simulink library "vmc"  (R2021b)
settings: Solver=VariableStepAuto  StartTime=0.0  StopTime=10.0  RelTol=1e-3
undefined symbols (not defined in the file or in its folder): AVMC_ACCDeltaTqIGain_X_kph, AVMC_ACCDeltaTqIGain_Y_mps2, AVMC_ACCDeltaTqPGain_X_kph, AVMC_ACCDeltaTqPGain_Y_kph, AVMC_ACCLongSteadyCtrl_X_kph, AVMC_AggressJerkPCT4AT_X_kph, AVMC_AggressJerkPCT_X_kph, AVMC_AggressLimitPCT4AT_X_kph, AVMC_AggressLimitPCT_X_kph, AVMC_CCLongSteadyCtrl_X_kph, AVMC_DISCDeltaTqIGain_X_kph, AVMC_DISCDeltaTqIGain_Y_mps2, AVMC_DISCDeltaTqPGain_X_kph, AVMC_DISCDeltaTqPGain_Y_kph, AVMC_DISCTrunAccJerk_X_s, AVMC_DISCTrunAccLimit_X_s, AVMC_ESCRegenOut_X_kph, AVMC_ESCRegenOut_Y_Deg, AVMC_ESCRegenOutEnSpd_X_Deg, AVMC_ISOAccLimit_X_mps, AVMC_ISODecLimit_X_mps, AVMC_ISOJerk_X_mps, AVMC_LatESCRegenOut_X_kph, AVMC_LatESCRegenOut_Y_Deg, AVMC_LongAccDeadZone_X_kph, AVMC_LongAccFiltTsforP2_X_Gps, AVMC_MCPresBaseTq_X_bar, AVMC_MSALongSteadyCtrl_X_kph, AVMC_MSAPedalOvrd2_X_kph, AVMC_MSAPedalOvrd_X_kph, AVMC_MSASpdBand_X_kph, AVMC_MSATqDownEndTq_X_kph, AVMC_MSATqDownTime_X_kph, AVMC_OPDDisSlideRate_X_Deg, AVMC_RDCDetectTime_X_kph, AVMC_RDCDetectTime_Y_pct, AVMC_RDCEnSlideRate_X_Deg, AVMC_RearWhlTqRatio_X_Nm, AVMC_RearWhlTqRatio_Y_gps, AVMC_RearWhlTqSlipGain_X_rat, AVMC_RearWhlTqSlipGain_Y_kph, AVMC_RearWhlTqSTRGGain_X_deg, AVMC_RearWhlTqSTRGGain_Y_kph, AVMC_RWSRrTSA2RWSPos_X_deg, AVMC_RWSSAS2FrtTSA_X_deg, AVMC_RWSVehSPD2RWSCoef_X_kph, AVMC_SoftJerkPCT_X_kph, AVMC_SoftLimitPCT_X_kph, AVMC_StESCYaw_X_kph, AVMC_StESCYaw_Y_Deg, AVMC_StESCYawCom_X_kph, AVMC_StESCYawCom_Y_Gps, AVMC_TMSpdBaseTq_X_rpm, AVMC_VehHoldBDecMap_X_kph, AVMC_VehHoldDecCtrlTime_X_kph, AVMC_VehHoldMCPPass_X_deg, C_TASK_10MS_S, C_TASK_5MS_S, DEG2RAD, ENUM_ACCAVAIL_AVAILABLE ... (+409)
libraries: hcu_lib x74, simulink x68, simulink_extras x3, $bdroot x2
(part 10 of 15)

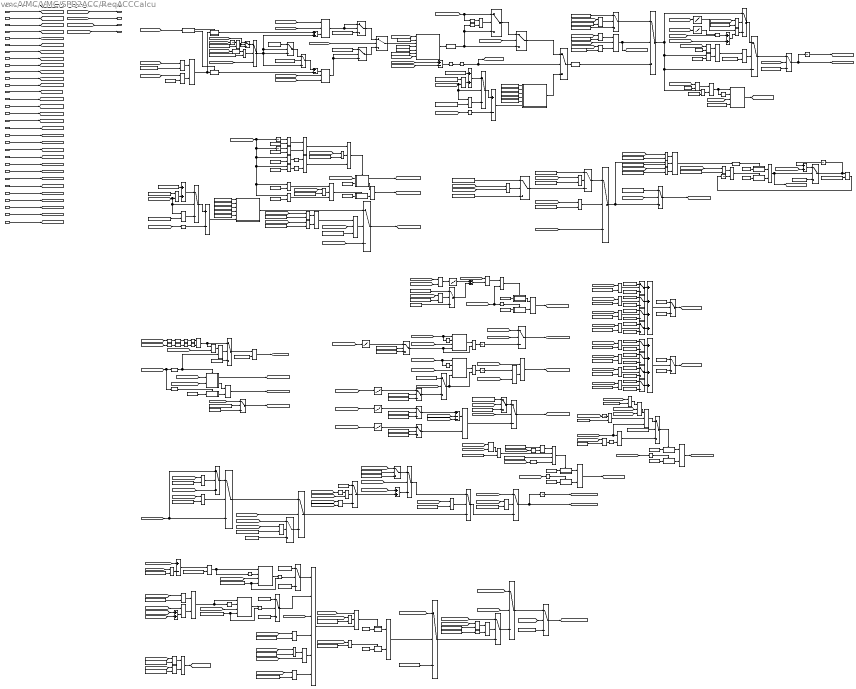
== system vmc/VMC/VMC/SPD2ACC/ReqACCCalcu ==
  note: FVT Soft Stop Control
      | (Send Hold Command after Reach H Time or ESC Standstill)
  note: Follow DISC Hold Time
      | (Avoid arbitrate error since CAN Signal sample time difference)
  note: Smooth Switch
      | (A, B-Pedal & REGEN to DISC)
  note: Required Acceleration for ESC
  note: Actual Required Acceleration
  note: DISC Required Acceleration
  note: Acceleration Arbitration
  note: ACC Speed Control
  note: Minimum Resolution
      | (Avoid too small command calculated from ISO Limit)
  note: Constant Speed Control
  note: Vehicle Hold Judgement and Command
  note: ACC Constant Speed Control
  note: ACC Constant Speed Control Judgement
  VVMC_AccCalcuPID_mps2 : Inport
  VVMC_ISOJerkLimit_mps3 : Inport  Port=2
  VVMC_JerkPCT_pct : Inport  Port=3
  VVMC_ISOAccLimit_mps2 : Inport  Port=4
  VVMC_ISODecLimit_mps2 : Inport  Port=5
  VVMC_SPD2ACCAct_flg : Inport  Port=6
  VVMC_SafetyCtrl_flg : Inport  Port=7
  VINP_ACCRequiredAccel_mps2 : Inport  Port=8
  VVMC_FeatArbitrSta_enum : Inport  Port=9
  VINP_ADASACCSta_enum : Inport  Port=10
  VVMC_MeterIndSpeedForCalcu_kph : Inport  Port=11
  VVMC_FeatReqSpd_kph : Inport  Port=12
  task_time_s : Inport  Port=13
  VINP_VehSpeed_kph : Inport  Port=14
  VVMC_LongAcc_Gps : Inport  Port=15
  VINP_ESCADASSta_enum : Inport  Port=16
  VVMC_LastADASWhlTqReq_Nm : Inport  Port=17
  VTQD_RrEDUAvailBrkRgnTq_Nm : Inport  Port=18
  VVMC_ACCVehHoldReq_flg : Inport  Port=19
  VVMC_EstSlope_Deg : Inport  Port=20
  VVMC_LongAccDeadZone_Gps : Inport  Port=21
  VTQD_FrEDUAvailBrkRgnTq_Nm : Inport  Port=22
  VVMC_ACCLowSpdTqCtrl_flg : Inport  Port=23
  VDSC_DISCTurn_flg : Inport  Port=24
  VINP_GRADE_Deg : Inport  Port=25
  VINP_LFWhlRotDir_enum : Inport  Port=26
  VINP_LRWhlRotDir_enum : Inport  Port=27
  VINP_RFWhlRotDir_enum : Inport  Port=28
  VINP_RRWhlRotDir_enum : Inport  Port=29
  VVMC_ACCObjDist_m : Inport  Port=30
  VINP_MCPressure_bar : Inport  Port=31
  VVMC_AccelTurnHold_flg : Inport  Port=32
  AND : Logic  Operator=OR  AllPortsSameDT=off  OutDataTypeStr=boolean
  AND{1,5..6,8..12,15} (9 alike) : Logic  AllPortsSameDT=off  OutDataTypeStr=boolean
  AND18 : Logic  Inputs=4  AllPortsSameDT=off  OutDataTypeStr=boolean
  AND2 : Logic  Inputs=3  AllPortsSameDT=off  OutDataTypeStr=boolean
  AND3 : Logic  Inputs=3  AllPortsSameDT=off  OutDataTypeStr=boolean
  AND4 : Logic  Inputs=3  AllPortsSameDT=off  OutDataTypeStr=boolean
  AND7 : Logic  Operator=OR  AllPortsSameDT=off  OutDataTypeStr=boolean
  Abs{,1..4} (5 alike) : Abs
  Add{,2,5,7,9} (5 alike) : Sum  Inputs=+-
  Add{1,3..4,6,8,11,14..15} (8 alike) : Sum
  Add10 : Sum  Inputs=+--
  Add12 : Sum  Inputs=++++
  Add13 : Sum  Inputs=++++
  CMDRepeat : Stateflow chart  TreatAsAtomicUnit=on
      settings: PortSchema="{\"entries\":[{\"content\":{\"sides\":[{\"content\":{\"connectorIds\":[\"In1\",\"In3\",\"In2\",\"In4\",\"In5\",\"In6\",\"In7\"]},\"type\":\"ConnectorPlacement.EquallySpacedRectSide\",\"uuid\":\"905b82c5-26d0-4d78-9cc9-ade9518b6cb1\"},{\"content\":{\"connectorIds\":[\"Out1\"],\"side\":\"RIGHT\"},\"type\":\"ConnectorPlacement.EquallySpacedRectSide\",\"uuid\":\"7321c4d8-dca0-41f9-ac80-faa74e816847\"},{\"content\":{\"connectorIds\":[],\"side\":\"TOP\"},\"type\":\"ConnectorPlacement.EquallySpacedRectSide\",\"uuid\":\"61a83612-f0ae-4eca-a4ee-e5180dc2049c\"}]},\"type\":\"ConnectorPlacement.EquallySpacedConnector\",\"uuid\":\"6863a8ab-8f7f-41d7-93f0-c1bbef1d5e3d\"}],\"packageUris\":[\"http://schema.mathworks.com/mf0/Connector/R2020b\"],\"version\":\"1.0\"}"
  Cast To Single{,1..2,7} (4 alike) : DataTypeConversion  OutDataTypeStr=single
  Constant : Constant  Value=pct
  Constant{1,7,19,27,34,39..40,42,44..45,49,64,66..68,78..79,81,89..93,95,112,115,125,127,129,131,139,141,143,145,157,163} (36 alike) : Constant  Value=ZERO_FLOAT
  Constant{10..12,17,20,32} (6 alike) : Constant  Value=ENUM_FEATARBITRSTA_DISC
  Constant100 : Constant  Value=KVMC_VehHoldDecCtrlBSlope4ATH_mps3
  Constant101 : Constant  Value=KVMC_ReqBrkJoinWaitTime_s
  Constant{50,52,70,102,106,108,134,148,150,153} (10 alike) : Constant  Value=FALSE
  Constant{48,51,69,94,97,103,107,109,111,133,147,154,161} (13 alike) : Constant  Value=TRUE
  Constant104 : Constant  Value=KVMC_AGSVReqAccel_mps2
  Constant105 : Constant  Value=KVMC_ReqBrkJoinWaitTime_s
  Constant110 : Constant  Value=KVMC_DISCTurnAccCtrl_flg
  Constant113 : Constant  Value=KVMC_DISCTurnAccSoftTime_s
  Constant114 : Constant  Value=KVMC_DISCTurnAccSoftTime_s
  Constant{117,122..124} (4 alike) : Constant  Value=ENUM_WheelRotDir_STANDSTILL
  Constant118 : Constant  Value=KVMC_VehHoldDelayHEndSW_flg
  Constant119 : Constant  Value=KVMC_VehHoldDist_m
  Constant121 : Constant  Value=KVMC_VehHoldDecCtrlCalSW2_flg
  Constant{30,126,128,130,132,140,142,144,146} (9 alike) : Constant  Value=ONE_FLOAT
  Constant{6,13,33,55,61} (5 alike) : Constant  Value=ENUM_FEATARBITRSTA_ACC
  Constant{135..138} (4 alike) : Constant  Value=ENUM_WheelRotDir_BACKWARD
  Constant14 : Constant  Value=KVMC_SpdCtrlEnBand_kph
  Constant149 : Constant  Value=KVMC_UpHillHoldDelayDeg_deg
  Constant15 : Constant  Value=KVMC_VehHoldDecCtrlBDec_mps2
  Constant151 : Constant  Value=KVMC_VehHoldDecCtrlBSlope_mps3
  Constant152 : Constant  Value=ENUM_FEATARBITRSTA_AEB
  Constant155 : Constant  Value=KVMC_DecCreepTq_Nm
  Constant156 : Constant  Value=KVMC_CreepTqMCP_bar
  Constant16 : Constant  Value=KVMC_Veh2MeterSpdFactor_enum
  Constant162 : Constant  Value=KVMC_VehHoldDecCtrlHTime2_s
  Constant18 : Constant  Value=KVMC_FollowDISCHoldTime_s
  Constant2 : Constant  Value=KVMC_CMDCycleTime_s
  Constant{5,8,21,56} (4 alike) : Constant  Value=ENUM_FEATARBITRSTA_ACCDISC
  Constant22 : Constant  Value=KVMC_AccelPos2NegSWC_flg
  Constant23 : Constant  Value=KVMC_Veh2MeterSpdOffset_enum
  Constant24 : Constant  Value=KVMC_SpdCtrlDisBand_kph
  Constant25 : Constant  Value=MINUSONE_FLOAT
  Constant26 : Constant  Value=KVMC_SpdCtrlReqAccel_mps2
  Constant28 : Constant  Value=KVMC_Veh2MeterSpdLoFactor_enum
  Constant29 : Constant  Value=KVMC_VehHoldSpd_kph
  Constant3 : Constant  Value=ZERO_INT
  Constant31 : Constant  Value=KVMC_VehHoldDecel_mps2
  Constant35 : Constant  Value=KVMC_SPD2ACCLastAccelSourceSW_flg
  Constant36 : Constant  Value=ENUM_ESCADASSTA_VEHASTANDSTILL
  Constant37 : Constant  Value=KVMC_GravityValue_mps2
  Constant{38,84..85,87,96} (5 alike) : Constant  Value=KVMC_VehHoldDecCtrlCalSW_flg
  Constant4 : Constant  Value=KVMC_CMDRepeatTime_enum
  Constant41 : Constant  Value=KVMC_GravityValue_mps2
  Constant43 : Constant  Value=KVMC_AccelCtrlTqLowerLimit_Nm
  Constant46 : Constant  Value=KVMC_SprtAccelCMDSW_flg
  Constant47 : Constant  Value=KVMC_TqAccelCtrlBand_mps2
  Constant53 : Constant  Value=KVMC_ReqAccelLowerLimit_mps2
  Constant54 : Constant  Value=KVMC_ReqDecelLowerLimit_mps2
  Constant57 : Constant  Value=KVMC_SpdCtrlEnBand_kph
  Constant58 : Constant  Value=KVMC_Veh2MeterSpdFactor_enum
  Constant59 : Constant  Value=KVMC_Veh2MeterSpdOffset_enum
  Constant60 : Constant  Value=KVMC_SpdCtrlDisBand_kph
  Constant62 : Constant  Value=MINUSONE_FLOAT
  Constant63 : Constant  Value=KVMC_SpdCtrlReqAccel_mps2
  Constant65 : Constant  Value=KVMC_Veh2MeterSpdLoFactor_enum
  Constant71 : Constant  Value=KVMC_ACCSpdCtrlSW_flg
  Constant72 : Constant  Value=ENUM_ADASACCSTA_OVERRIDE
  Constant73 : Constant  Value=ENUM_ADASACCSTA_OVERRIDE
  Constant74 : Constant  Value=KVMC_VehHoldDecCtrl_flg
  Constant75 : Constant  Value=KVMC_VehHoldDecCtrlBTime_s
  Constant76 : Constant  Value=KVMC_VehHoldDecCtrlBDec_mps2
  Constant77 : Constant  Value=KVMC_GravityValue_mps2
  Constant80 : Constant  Value=KVMC_VehHoldDecCtrlBTime_s
  Constant82 : Constant  Value=KVMC_CallBrkJoinSpd_kph
  Constant83 : Constant  Value=KVMC_VehHoldDecCtrlHTime_s
  Constant86 : Constant  Value=ENUM_ADASACCSTA_ACTIVE
  Constant88 : Constant  Value=KVMC_VehHoldDecCtrlGFBSW_flg
  Constant9 : Constant  Value=ENUM_ADASACCSTA_OVERRIDE
  Constant98 : Constant  Value=KVMC_AccelTurnHoldDecCtrl2_flg
  Constant99 : Constant  Value=ENUM_ADASACCSTA_ACTIVE
  ConstantSpeedControl : Stateflow chart  TreatAsAtomicUnit=on
      settings: PortSchema="{\"entries\":[{\"content\":{\"sides\":[{\"content\":{\"connectorIds\":[\"In2\",\"In3\",\"In4\",\"In5\",\"In6\",\"In1\"]},\"type\":\"ConnectorPlacement.EquallySpacedRectSide\",\"uuid\":\"931d4d55-b643-4b97-a7aa-1deb2b509e83\"},{\"content\":{\"connectorIds\":[\"Out1\"],\"side\":\"RIGHT\"},\"type\":\"ConnectorPlacement.EquallySpacedRectSide\",\"uuid\":\"f2f28b13-6937-4f35-b44e-683edec0d4ba\"},{\"content\":{\"connectorIds\":[],\"side\":\"TOP\"},\"type\":\"ConnectorPlacement.EquallySpacedRectSide\",\"uuid\":\"e2886b86-de2a-4a68-b05f-bfb0f2051baf\"}]},\"type\":\"ConnectorPlacement.EquallySpacedConnector\",\"uuid\":\"cece4c76-e980-42e8-adab-da09fec387c1\"}],\"packageUris\":[\"http://schema.mathworks.com/mf0/Connector/R2020b\"],\"version\":\"1.0\"}"
  ConstantSpeedControl1 : Stateflow chart  TreatAsAtomicUnit=on
      settings: PortSchema="{\"entries\":[{\"content\":{\"sides\":[{\"content\":{\"connectorIds\":[\"In2\",\"In3\",\"In4\",\"In5\",\"In6\",\"In1\"]},\"type\":\"ConnectorPlacement.EquallySpacedRectSide\",\"uuid\":\"931d4d55-b643-4b97-a7aa-1deb2b509e83\"},{\"content\":{\"connectorIds\":[\"Out1\"],\"side\":\"RIGHT\"},\"type\":\"ConnectorPlacement.EquallySpacedRectSide\",\"uuid\":\"f2f28b13-6937-4f35-b44e-683edec0d4ba\"},{\"content\":{\"connectorIds\":[],\"side\":\"TOP\"},\"type\":\"ConnectorPlacement.EquallySpacedRectSide\",\"uuid\":\"e2886b86-de2a-4a68-b05f-bfb0f2051baf\"}]},\"type\":\"ConnectorPlacement.EquallySpacedConnector\",\"uuid\":\"cece4c76-e980-42e8-adab-da09fec387c1\"}],\"packageUris\":[\"http://schema.mathworks.com/mf0/Connector/R2020b\"],\"version\":\"1.0\"}"
  Degrees to Radians1 : simulink_extras/Transformations/Degrees to Radians
  Degrees to Radians2 : simulink_extras/Transformations/Degrees to Radians
  Detect Decrease : simulink/Logic and Bit Operations/Detect Decrease  vinit=0.0  OutDataTypeStr=boolean
  Detect Increase{,1..2,5} (4 alike) : simulink/Logic and Bit Operations/Detect Increase  vinit=0.0  OutDataTypeStr=boolean
  Divide : Product  Inputs=*/
  Divide{1..3,5,8..12,16} (10 alike) : Product  Inputs=**
  Divide13 : Product  Inputs=*/
  Divide14 : Product  Inputs=*/
  If Action Subsystem4 : Subsystem  TreatAsAtomicUnit=on
  If Action Subsystem5 : Subsystem  TreatAsAtomicUnit=on
  If1 : If
  InitialCondition: 0 : UnitDelay  SampleTime=-1  HasFrameUpgradeWarning=on
  InitialCondition: 0 (1) : UnitDelay  SampleTime=-1  HasFrameUpgradeWarning=on
  Logical Operator : Logic  Inputs=3  AllPortsSameDT=off  OutDataTypeStr=boolean
  Logical Operator1 : Logic  Inputs=3  AllPortsSameDT=off  OutDataTypeStr=boolean
  Logical Operator2 : Logic  Operator=OR  Inputs=6  AllPortsSameDT=off  OutDataTypeStr=boolean
  Logical Operator4 : Logic  AllPortsSameDT=off  OutDataTypeStr=boolean
  Logical Operator5 : Logic  Operator=OR  AllPortsSameDT=off  OutDataTypeStr=boolean
  MVMC_DISCTrunAccJerk_Y_mps3 : Lookup_n-D  NumberOfTableDimensions=1  BreakpointsForDimension1=AVMC_DISCTrunAccJerk_X_s  Table=MVMC_DISCTrunAccJerk_Y_mps3  InterpMethod=Flat  InternalRulePriority=Speed  RndMeth=Simplest  InputSameDT=on
  MVMC_DISCTrunAccLimit_Y_mps2 : Lookup_n-D  NumberOfTableDimensions=1  BreakpointsForDimension1=AVMC_DISCTrunAccLimit_X_s  Table=MVMC_DISCTrunAccLimit_Y_mps2  InternalRulePriority=Speed  RndMeth=Simplest  InputSameDT=on
  MVMC_VehHoldBDecMap_Y_mps2 : Lookup_n-D  NumberOfTableDimensions=1  BreakpointsForDimension1=AVMC_VehHoldBDecMap_X_kph  Table=MVMC_VehHoldBDecMap_Y_mps2  InternalRulePriority=Speed  RndMeth=Simplest  InputSameDT=on
  MVMC_VehHoldDecCtrlTime_Y_s : Lookup_n-D  NumberOfTableDimensions=1  BreakpointsForDimension1=AVMC_VehHoldDecCtrlTime_X_kph  Table=MVMC_VehHoldDecCtrlTime_Y_s  InternalRulePriority=Speed  RndMeth=Simplest  InputSameDT=on
  MVMC_VehHoldDecCtrlTime_Y_s1 : Lookup_n-D  NumberOfTableDimensions=1  BreakpointsForDimension1=AVMC_VehHoldDecCtrlTime_X_kph  Table=MVMC_VehHoldDecCtrlTime_Y_s  InternalRulePriority=Speed  RndMeth=Simplest  InputSameDT=on
  MVMC_VehHoldDecCtrlTime_Y_s2 : Lookup_n-D  NumberOfTableDimensions=1  BreakpointsForDimension1=AVMC_VehHoldDecCtrlTime_X_kph  Table=MVMC_VehHoldDecCtrlTime_Y_s  InternalRulePriority=Speed  RndMeth=Simplest  InputSameDT=on
  MVMC_VehHoldMCPPass_Y_bar : Lookup_n-D  NumberOfTableDimensions=1  BreakpointsForDimension1=AVMC_VehHoldMCPPass_X_deg  Table=MVMC_VehHoldMCPPass_Y_bar  InternalRulePriority=Speed  RndMeth=Simplest  InputSameDT=on
  Max : MinMax  Function=max  Inputs=2
  Max4 : MinMax  Function=max  Inputs=2
  Max5 : MinMax  Function=max  Inputs=2
  Merge{,1..6} (7 alike) : Merge
  Min : MinMax  Inputs=2
  MinMax2 : MinMax  Inputs=3
  MinMax3 : MinMax  Function=max  Inputs=3
  NOT{,1..12,14} (14 alike) : Logic  Operator=NOT  AllPortsSameDT=off  OutDataTypeStr=boolean
  OR{,1..4,9} (6 alike) : Logic  Operator=OR  AllPortsSameDT=off  OutDataTypeStr=boolean
  OR5 : Logic  AllPortsSameDT=off  OutDataTypeStr=boolean
  OR6 : Logic  Operator=OR  Inputs=3  AllPortsSameDT=off  OutDataTypeStr=boolean
  OR7 : Logic  Operator=OR  Inputs=3  AllPortsSameDT=off  OutDataTypeStr=boolean
  OR8 : Logic  Inputs=3  AllPortsSameDT=off  OutDataTypeStr=boolean
  Relational Operator{,7,15..16,18,31,41,48} (8 alike) : RelationalOperator  Operator=<=  OutDataTypeStr=boolean  RndMeth=Simplest
  Relational Operator{1..5,8,10,12..14,21..23,28,33,37,44,49..56,59} (26 alike) : RelationalOperator  Operator===  OutDataTypeStr=boolean  RndMeth=Simplest
  Relational Operator{6,11,20,24..25,35,58,62} (8 alike) : RelationalOperator  Operator=<  OutDataTypeStr=boolean  RndMeth=Simplest
  Relational Operator{9,17,19,29..30,32,40,42,46,57,61} (11 alike) : RelationalOperator  OutDataTypeStr=boolean  RndMeth=Simplest
  Relational Operator{26,34,36,43,45,47} (6 alike) : RelationalOperator  Operator=>  OutDataTypeStr=boolean  RndMeth=Simplest
  Relational Operator27 : RelationalOperator  Operator=~=  OutDataTypeStr=boolean  RndMeth=Simplest
  Relational Operator38 : RelationalOperator  Operator=~=  OutDataTypeStr=boolean  RndMeth=Simplest
  Round : Rounding  Operator=round
  Round3 : Rounding  Operator=round
  Round4 : Rounding  Operator=round
  Sin1 : Trigonometry
  Sin2 : Trigonometry
  Switch : Switch  Criteria=u2 > Threshold  Threshold=KVMC_Veh2MeterSpdLoBdy_kph
  Switch1 : Switch  Criteria=u2 > Threshold  Threshold=KVMC_Veh2MeterSpdLoBdy_kph
  Switch{2..18,20..21,23..25,27..30,33..35} (29 alike) : Switch  Criteria=u2 > Threshold
  Switch26 : Switch  Threshold=TWO_FLOAT
  Switch31 : Switch  Threshold=TWO_FLOAT
  Timer{,1..4} (5 alike) : hcu_lib/Basic_Blocks/Timer
  Triggered Subsystem : Subsystem  TreatAsAtomicUnit=on
  Triggered Subsystem1 : Subsystem  TreatAsAtomicUnit=on
  Triggered Subsystem10 : Subsystem  TreatAsAtomicUnit=on
  Triggered Subsystem11 : Subsystem  TreatAsAtomicUnit=on
  Triggered Subsystem12 : Subsystem  TreatAsAtomicUnit=on
  Triggered Subsystem13 : Subsystem  TreatAsAtomicUnit=on
  Triggered Subsystem2 : Subsystem  TreatAsAtomicUnit=on
  Triggered Subsystem3 : Subsystem  TreatAsAtomicUnit=on
  Triggered Subsystem4 : Subsystem  TreatAsAtomicUnit=on
  Triggered Subsystem5 : Subsystem  TreatAsAtomicUnit=on
  Triggered Subsystem6 : Subsystem  TreatAsAtomicUnit=on
  Triggered Subsystem7 : Subsystem  TreatAsAtomicUnit=on
  Triggered Subsystem8 : Subsystem  TreatAsAtomicUnit=on
  Triggered Subsystem9 : Subsystem  TreatAsAtomicUnit=on
  Unit Delay{,1..5,9} (7 alike) : UnitDelay  SampleTime=-1  HasFrameUpgradeWarning=on
  initial = 0 (2) : UnitDelay  SampleTime=-1  HasFrameUpgradeWarning=on
  u2 > 0 (1){,1..9} (10 alike) : Switch  Criteria=u2 > Threshold
  u2 > 0 (10) : Switch  Criteria=u2 > Threshold
  u2 > 0 (11) : Switch  Criteria=u2 > Threshold
  u2 > 0 (13) : Switch  Criteria=u2 > Threshold
  u2 > 0 (14) : Switch  Criteria=u2 > Threshold
  u2 > 0 (16) : Switch  Criteria=u2 > Threshold
  u2 > 0 (16)1 : Switch  Criteria=u2 > Threshold  Threshold=KVMC_ReqAccelLowerLimit_mps2
  u2 > 0 (16)2 : Switch  Criteria=u2 > Threshold  Threshold=KVMC_ReqDecelLowerLimit_mps2
  u2 > 0 (2) : Switch  Criteria=u2 > Threshold
  u2 > 0 (3) : Switch  Criteria=u2 > Threshold
  u2 > 0 (3)2 : Switch  Criteria=u2 > Threshold
  u2 > 0 (4) : Switch  Criteria=u2 > Threshold
  u2 > 0 (5) : Switch  Criteria=u2 > Threshold
  u2 > 0 (6) : Switch  Criteria=u2 > Threshold
  u2 > 0 (7) : Switch  Criteria=u2 > Threshold
  u2 > 0 (8) : Switch  Criteria=u2 > Threshold
  u2 > 0 (9) : Switch  Criteria=u2 > Threshold
  u2 >= 0 : Switch
  "VVMC_ACCRequiredAccel_mps2 " : Outport
  VVMC_FeatArbitrFinal_enum : Outport  Port=2
  VVMC_VehHoldReq_flg : Outport  Port=3
  VVMC_ActACCRequiredAccel_mps2 : Outport  Port=4
  VVMC_VehHoldDecCtrlHEnd_flg : Outport  Port=5
  wires:
  Switch7/1 -> InitialCondition: 0 (1)/1, [VVMC_DISCReqAcc_mps2]  "VVMC_DISCReqAcc_mps2"
  Constant22/1 -> u2 > 0 (16)/2
  u2 > 0 (16)/1 -> Add/1
  [VVMC_DISCReqAcc_mps2] -> u2 > 0 (9)/1, u2 > 0 (2)/3
  Relational Operator5/1 -> u2 > 0 (9)/2
  [VVMC_AfterCtrlACCReqAccel_mps2] -> u2 > 0 (9)/3
  InitialCondition: 0/1 -> [VVMC_LastActACCRequiredAccel_mps2]  "VVMC_LastActACCRequiredAccel_mps2"
  u2 > 0 (5)/1 -> u2 > 0 (1)/3
  u2 > 0 (2)/1 -> u2 > 0 (1)/1
  [VVMC_SPD2ACCAct_flg] -> u2 > 0 (1)/2
  [VVMC_FeatArbitrSta_enum] -> Relational Operator1/1
  [VVMC_FeatArbitrSta_enum] -> Relational Operator2/1
  Constant1/1 -> u2 > 0 (5)/3
  Constant11/1 -> Relational Operator5/2
  Constant5/1 -> Relational Operator1/2
  Relational Operator1/1 -> u2 > 0 (2)/2
  Constant6/1 -> Relational Operator2/2
  u2 > 0 (9)/1 -> u2 > 0 (2)/1
  Relational Operator2/1 -> u2 > 0 (5)/2
  [VVMC_AfterCtrlACCReqAccel_mps2] -> u2 > 0 (5)/1
  u2 > 0 (1)9/1 -> [VVMC_ActACCRequiredAccel_mps2], InitialCondition: 0/1  "VVMC_ActACCRequiredAccel_mps2"
  [VVMC_FeatArbitrFinal_enum] -> Relational Operator5/1
  Cast To Single7/1 -> u2 > 0 (3)/3, u2 > 0 (4)/3, Abs1/1
  [VVMC_SafetyCtrl_flg] -> u2 > 0 (3)/2
  Abs/1 -> Relational Operator/1
  Relational Operator/1 -> u2 > 0 (4)/2
  [VVMC_LastActACCRequiredAccel_mps2] -> Abs/1, u2 > 0 (4)/1
  Abs1/1 -> Relational Operator/2
  u2 > 0 (4)/1 -> u2 > 0 (3)/1
  Relational Operator10/1 -> Logical Operator/1
  Constant17/1 -> Relational Operator8/2
  Relational Operator8/1 -> Logical Operator/2
  Constant21/1 -> Relational Operator10/2
  [VVMC_FeatArbitrSta_enum] -> Relational Operator10/1
  Constant20/1 -> u2 > 0 (14)/1
  Constant19/1 -> u2 > 0 (13)/3
  Constant18/1 -> Relational Operator9/2
  Add3/1 -> u2 > 0 (13)/1
  u2 > 0 (13)/1 -> Relational Operator9/1, initial = 0 (2)/1
  [task_time_s] -> Add3/2
  Logical Operator/1 -> Detect Increase1/1
  u2 > 0 (7)/1 -> Relational Operator8/1, u2 > 0 (14)/3
  task_time_s/1 -> [task_time_s]
  [VVMC_MeterIndSpeedForCalcu_kph] -> Add2/2
  [VVMC_FeatReqSpd_kph] -> Add2/1
  u2 > 0 (11)/1 -> Cast To Single1/1
  Round/1 -> [VVMC_AbsDeltaSpd_kph], u2 > 0 (11)/2
  Abs2/1 -> Round/1
  Add2/1 -> Abs2/1
  VVMC_MeterIndSpeedForCalcu_kph/1 -> [VVMC_MeterIndSpeedForCalcu_kph]
  VVMC_FeatReqSpd_kph/1 -> [VVMC_FeatReqSpd_kph]
  u2 > 0 (3)/1 -> u2 > 0 (11)/1
  InitialCondition: 0 (1)/1 -> [VVMC_LastDISCReqAcc_mps2]  "VVMC_LastDISCReqAcc_mps2"
  Constant13/1 -> u2 > 0 (10)/1
  Constant12/1 -> u2 > 0 (10)/3
  u2 > 0 (10)/1 -> u2 > 0 (8)/3
  Relational Operator6/1 -> u2 > 0 (10)/2
  Constant10/1 -> u2 > 0 (8)/1
  Relational Operator4/1 -> u2 > 0 (8)/2
  [VVMC_AfterCtrlACCReqAccel_mps2] -> Relational Operator6/1
  [VVMC_DISCReqAcc_mps2] -> Relational Operator6/2
  [VINP_ADASACCSta_enum] -> Relational Operator4/1
  Constant9/1 -> Relational Operator4/2
  VINP_ADASACCSta_enum/1 -> [VINP_ADASACCSta_enum]
  [VVMC_FeatArbitrFinal_enum] -> VVMC_FeatArbitrFinal_enum/1
  u2 > 0 (14)/1 -> [VVMC_FeatArbitrFinal_enum]  "VVMC_FeatArbitrFinal_enum"
  [VVMC_FeatArbitrSta_enum] -> u2 > 0 (7)/3
  u2 > 0 (8)/1 -> u2 > 0 (7)/1
  Relational Operator3/1 -> u2 > 0 (7)/2
  [VVMC_FeatArbitrSta_enum] -> Relational Operator3/1
  Constant8/1 -> Relational Operator3/2
  u2 > 0 (6)/1 -> u2 > 0 (16)/1
  Constant7/1 -> u2 > 0 (6)/1
  VVMC_FeatArbitrSta_enum/1 -> [VVMC_FeatArbitrSta_enum]
  VINP_ACCRequiredAccel_mps2/1 -> [VINP_ACCRequiredAccel_mps2]
  VVMC_SafetyCtrl_flg/1 -> [VVMC_SafetyCtrl_flg]
  Constant4/1 -> CMDRepeat/6(KVMC_CMDRepeatTime_enum)
  Constant3/1 -> CMDRepeat/5(ZERO_INT)
  [VVMC_ACCRequiredAccel_mps2] -> "VVMC_ACCRequiredAccel_mps2 "/1
  Add1/1 -> MinMax2/3
  Constant2/1 -> Divide1/2
  [VVMC_ISOJerkLimit_mps3] -> Divide1/1
  Constant/1 -> Divide/2
  VVMC_SPD2ACCAct_flg/1 -> [VVMC_SPD2ACCAct_flg]
  VVMC_ISODecLimit_mps2/1 -> [VVMC_ISODecLimit_mps2]
  VVMC_ISOAccLimit_mps2/1 -> [VVMC_ISOAccLimit_mps2]
  VVMC_JerkPCT_pct/1 -> [VVMC_JerkPCT_pct]
  VVMC_ISOJerkLimit_mps3/1 -> [VVMC_ISOJerkLimit_mps3]
  VVMC_AccCalcuPID_mps2/1 -> [VVMC_AccCalcuPID_mps2]
  Switch2/1 -> u2 > 0 (6)/2, Add1/2, u2 > 0 (16)/3, u2 > 0 (6)/3
  [VVMC_AccCalcuPID_mps2] -> u2 >= 0/2
  [VVMC_AccCalcuPID_mps2] -> MinMax3/3
  [VVMC_AccCalcuPID_mps2] -> MinMax2/1
  [VVMC_JerkPCT_pct] -> Divide/1
  Divide1/1 -> Divide2/1
  If1/2 -> If Action Subsystem5/Action
  If Action Subsystem5/1(Out1) -> Add/2
  [VVMC_ISODecLimit_mps2] -> MinMax3/2
  [VVMC_AccCalcuPID_mps2] -> If1/1
  If Action Subsystem4/1(Out1) -> Add1/1
  MinMax2/1 -> u2 > 0 (16)1/1, u2 > 0 (16)1/2
  [VVMC_ISOAccLimit_mps2] -> MinMax2/2
  Divide/1 -> Divide2/2
  Divide2/1 -> If Action Subsystem5/1(In1), If Action Subsystem4/1(In1)
  u2 >= 0/1 -> CMDRepeat/2(VVMC_ReqAccCalcu_mps2)
  If1/1 -> If Action Subsystem4/Action
  CMDRepeat/1(VVMC_ReqAcc_mps2) -> Cast To Single7/1
  Add/1 -> MinMax3/1
  VINP_VehSpeed_kph/1 -> [VINP_VehSpeed_kph]
  Divide5/1 -> Add4/2
  [VINP_VehSpeed_kph] -> Switch/2, Divide8/1, Divide5/2
  Constant23/1 -> Add4/1
  Constant16/1 -> Divide5/1
  Add4/1 -> Switch/1
  Round3/1 -> Add5/2
  Add5/1 -> ConstantSpeedControl/1(DeltaSpeed)
  Constant14/1 -> ConstantSpeedControl/2(KVMC_SpdCtrlEnBand_kph)
  Constant24/1 -> ConstantSpeedControl/3(KVMC_SpdCtrlDisBand_kph)
  Constant25/1 -> ConstantSpeedControl/4(MINUSONE_FLOAT)
  [VVMC_FeatReqSpd_kph] -> Round3/1
  Constant26/1 -> ConstantSpeedControl/5(KVMC_SpdCtrlReqAccel_mps2)
  Constant27/1 -> ConstantSpeedControl/6(ZERO_FLOAT)
  Divide8/1 -> Switch/3
  Constant28/1 -> Divide8/2
  Switch/1 -> Add5/1
  ConstantSpeedControl/1(ReqAccel) -> u2 > 0 (11)/3
  [VVMC_SPD2ACCAct_flg] -> Detect Increase/1
  VVMC_LongAcc_Gps/1 -> [VVMC_LongAcc_Gps]
  Constant35/1 -> Logical Operator4/2
  Detect Increase/1 -> Logical Operator4/1
  Logical Operator4/1 -> Switch2/2
  [VVMC_LastDISCReqAcc_mps2] -> Switch2/3
  [VVMC_LastDISCReqAcc_mps2] -> Switch6/1
  Divide9/1 -> Switch6/3, Switch6/2
  [VVMC_LongAcc_Gps] -> Unit Delay1/1
  Constant37/1 -> Divide9/2
  Switch6/1 -> Switch2/1
  Cast To Single1/1 -> u2 > 0 (3)2/3
  Logical Operator1/1 -> u2 > 0 (3)2/2, [VVMC_VehHoldReq_flg]
  Constant36/1 -> Relational Operator12/2
  [VINP_ESCADASSta_enum] -> Relational Operator12/1
  [VINP_VehSpeed_kph] -> Relational Operator7/1
  Relational Operator11/1 -> Logical Operator1/3
  Constant29/1 -> Relational Operator7/2
  Constant40/1 -> Switch4/1
  [VVMC_SPD2ACCAct_flg] -> Switch7/2
  Relational Operator7/1 -> Logical Operator1/1
  Constant30/1 -> Relational Operator11/2
  [VVMC_SPD2ACCAct_flg] -> Logical Operator1/2
  Relational Operator12/1 -> Switch4/2
  Constant31/1 -> Switch4/3
  Switch16/1 -> Switch7/1
  [VVMC_FeatReqSpd_kph] -> Relational Operator11/1
  Constant42/1 -> Switch7/3
  Switch4/1 -> u2 > 0 (3)2/1
  VINP_ESCADASSta_enum/1 -> [VINP_ESCADASSta_enum]
  Triggered Subsystem/1(Out1) -> Merge1/1
  Constant52/1 -> Triggered Subsystem1/1(In1)
  Constant49/1 -> Relational Operator19/2
  Constant45/1 -> u2 > 0 (1)1/3
  Logical Operator2/1 -> AND2/3
  [VVMC_ActACCRequiredAccel_mps2] -> u2 > 0 (1)1/1
  Triggered Subsystem1/1(Out1) -> Merge1/2
  [VVMC_LongAcc_Gps] -> Divide10/1
  Constant47/1 -> Relational Operator18/2
  [VVMC_ActACCRequiredAccel_mps2] -> Relational Operator19/1
  Constant44/1 -> Relational Operator17/2
  Relational Operator17/1 -> AND/1
  [VVMC_LastADASWhlTqReq_Nm] -> Relational Operator15/1
  u2 > 0 (1)1/1 -> u2 > 0 (1)3/3
  Constant46/1 -> NOT/1
  NOT/1 -> AND/2
  AND/1 -> u2 > 0 (1)3/2
  Relational Operator15/1 -> Logical Operator5/2
  [VTQD_RrEDUAvailBrkRgnTq_Nm] -> Add14/1
  Relational Operator16/1 -> Logical Operator5/1
  Constant43/1 -> Relational Operator16/2
  Constant51/1 -> Triggered Subsystem/1(In1)
  [VVMC_ActACCRequiredAccel_mps2] -> Relational Operator17/1
  [VVMC_ActACCRequiredAccel_mps2] -> u2 > 0 (1)2/1
  [VVMC_ACCVehHoldReq_flg] -> u2 > 0 (1)2/2
  Add7/1 -> Relational Operator18/1
  [VVMC_ActACCRequiredAccel_mps2] -> Add7/1
  Merge1/1 -> u2 > 0 (1)1/2  "VVMC_ReqBrkJoin_flg"
  u2 > 0 (1)3/1 -> u2 > 0 (1)2/3
  [VVMC_LastADASWhlTqReq_Nm] -> Relational Operator16/1
  Divide10/1 -> Add7/2
  Constant41/1 -> Divide10/2
  [VVMC_ActACCRequiredAccel_mps2] -> u2 > 0 (1)3/1
  u2 > 0 (1)4/1 -> [VVMC_ACCRequiredAccel_mps2]
  Relational Operator13/1 -> OR/1
  Constant32/1 -> Relational Operator13/2
  Constant33/1 -> Relational Operator14/2
  OR/1 -> [VVMC_ReqAccelActive_flg]
  [VVMC_FeatArbitrFinal_enum] -> Relational Operator13/1
  [VVMC_FeatArbitrFinal_enum] -> Relational Operator14/1
  Relational Operator14/1 -> OR/2
  [VVMC_ReqAccelActive_flg] -> u2 > 0 (1)4/2
  u2 > 0 (1)2/1 -> u2 > 0 (1)4/1
  Constant34/1 -> u2 > 0 (1)4/3
  Relational Operator19/1 -> Triggered Subsystem1/Trigger
  [VVMC_ReqAccelActive_flg] -> AND2/1
  AND2/1 -> Triggered Subsystem/Trigger
  [VVMC_ActACCRequiredAccel_mps2] -> Relational Operator20/1
  Constant39/1 -> Relational Operator20/2
  Relational Operator20/1 -> AND2/2
  Detect Increase1/1 -> Triggered Subsystem2/Trigger
  Constant48/1 -> Triggered Subsystem2/1(In1)
  Triggered Subsystem2/1(Out1) -> Merge/1
  Triggered Subsystem3/1(Out1) -> Merge/2
  Constant50/1 -> Triggered Subsystem3/1(In1)
  Relational Operator9/1 -> Unit Delay/1
  Merge/1 -> u2 > 0 (13)/2, [VVMC_FollowDISCHoldSta_flg]  "VVMC_FollowDISCHoldSta_flg"
  initial = 0 (2)/1 -> Add3/1
  Unit Delay/1 -> OR2/2
  VTQD_RrEDUAvailBrkRgnTq_Nm/1 -> [VTQD_RrEDUAvailBrkRgnTq_Nm]
  VVMC_LastADASWhlTqReq_Nm/1 -> [VVMC_LastADASWhlTqReq_Nm]
  [VVMC_ActACCRequiredAccel_mps2] -> VVMC_ActACCRequiredAccel_mps2/1
  [VVMC_VehHoldReq_flg] -> VVMC_VehHoldReq_flg/1  "VVMC_VehHoldReq_flg"
  Constant53/1 -> u2 > 0 (16)1/3
  u2 > 0 (16)1/1 -> u2 >= 0/1
  Constant54/1 -> u2 > 0 (16)2/1
  MinMax3/1 -> u2 > 0 (16)2/3, u2 > 0 (16)2/2
  u2 > 0 (16)2/1 -> u2 >= 0/3
  Unit Delay1/1 -> Divide9/1
  AND1/1 -> Logical Operator2/5
  Relational Operator21/1 -> AND1/1
  [VVMC_FeatArbitrFinal_enum] -> Relational Operator21/1
  Constant61/1 -> Relational Operator21/2
  [VVMC_SafetyCtrl_flg] -> AND1/2
  Constant55/1 -> Relational Operator22/2
  [VVMC_FeatArbitrSta_enum] -> Relational Operator22/1
  Constant56/1 -> Relational Operator23/2
  [VVMC_FeatArbitrSta_enum] -> Relational Operator23/1
  Relational Operator23/1 -> OR1/1
  Relational Operator22/1 -> OR1/2
  Constant58/1 -> Divide11/1
  [VINP_VehSpeed_kph] -> Switch1/2, Divide12/1, Divide11/2
  Divide11/1 -> Add8/2
  Constant65/1 -> Divide12/2
  ConstantSpeedControl1/1(ReqAccel) -> Switch5/1
  Add9/1 -> ConstantSpeedControl1/1(DeltaSpeed)
  Constant63/1 -> ConstantSpeedControl1/5(KVMC_SpdCtrlReqAccel_mps2)
  Constant64/1 -> ConstantSpeedControl1/6(ZERO_FLOAT)
  [VVMC_ACCReqSpdMemory_kph] -> Round4/1
  Constant60/1 -> ConstantSpeedControl1/3(KVMC_SpdCtrlDisBand_kph)
  Switch1/1 -> Add9/1
  Divide12/1 -> Switch1/3
  Constant59/1 -> Add8/1
  Add8/1 -> Switch1/1
  Constant57/1 -> ConstantSpeedControl1/2(KVMC_SpdCtrlEnBand_kph)
  Round4/1 -> Add9/2
  Constant62/1 -> ConstantSpeedControl1/4(MINUSONE_FLOAT)
  Unit Delay2/1 -> Relational Operator24/1
  Constant66/1 -> Relational Operator24/2
  OR5/1 -> AND3/3
  Relational Operator24/1 -> OR4/1
  AND3/1 -> Triggered Subsystem4/Trigger
  Triggered Subsystem4/1(Out1) -> [VVMC_ACCReqSpdMemory_kph]  "VVMC_ACCReqSpdMemory_kph"
  Constant69/1 -> Triggered Subsystem4/2(In2)
  Triggered Subsystem4/2(Out2) -> Merge2/1
  OR6/1 -> Triggered Subsystem5/Trigger
  Constant70/1 -> Triggered Subsystem5/1(In1)
  Triggered Subsystem5/1(Out1) -> Merge2/2
  Merge2/1 -> [VVMC_ACCSpdCtrl_flg]  "VVMC_ACCSpdCtrl_flg"
  OR1/1 -> AND4/1
  [VVMC_ACCSpdCtrl_flg] -> AND4/2
  Constant71/1 -> AND4/3
  AND4/1 -> Switch5/2
  [VINP_ACCRequiredAccel_mps2] -> Switch5/3
  Switch5/1 -> [VVMC_AfterCtrlACCReqAccel_mps2]  "VVMC_AfterCtrlACCReqAccel_mps2"
  Constant72/1 -> Relational Operator27/2
  [VINP_ADASACCSta_enum] -> Relational Operator27/1
  Relational Operator27/1 -> Logical Operator/3
  [VVMC_FollowDISCHoldSta_flg] -> u2 > 0 (14)/2
  [VINP_ADASACCSta_enum] -> Relational Operator28/1
  Constant73/1 -> Relational Operator28/2
  Relational Operator28/1 -> OR2/1
  OR2/1 -> Triggered Subsystem3/Trigger
  VVMC_ACCVehHoldReq_flg/1 -> [VVMC_ACCVehHoldReq_flg]
  [VVMC_ACCVehHoldReq_flg] -> AND5/1
  u2 > 0 (1)/1 -> u2 > 0 (1)5/3
  Constant74/1 -> AND5/2
  AND5/1 -> u2 > 0 (1)5/2
  Cast To Single/1 -> Sin1/1
  Degrees to Radians1/1 -> Cast To Single/1
  Sin1/1 -> Abs4/1
  VVMC_EstSlope_Deg/1 -> [VVMC_EstSlope_Deg]
  [VVMC_EstSlope_Deg] -> Degrees to Radians1/1
  Abs4/1 -> Max/2
  Constant77/1 -> Divide13/2
  VVMC_LongAccDeadZone_Gps/1 -> [VVMC_LongAccDeadZone_Gps]
  [VVMC_LongAccDeadZone_Gps] -> Relational Operator29/2
  Relational Operator29/1 -> AND6/1
  Constant78/1 -> Switch8/3
  Switch8/1 -> Divide13/1
  Divide13/1 -> [VVMC_BrkGFB_mps2]  "VVMC_BrkGFB_mps2"
  [VVMC_ACCVehHoldReq_flg] -> Detect Decrease/1, Detect Increase2/1
  Detect Increase2/1 -> AND6/2, Triggered Subsystem6/Trigger
  [VVMC_LastActACCRequiredAccel_mps2] -> Triggered Subsystem6/2(In2)
  Merge3/1 -> [VVMC_VehHoldEnReqAccel_mps2]  "VVMC_VehHoldEnReqAccel_mps2"
  Constant79/1 -> Triggered Subsystem7/1(In1)
  Detect Decrease/1 -> Triggered Subsystem7/Trigger
  Triggered Subsystem6/2(Out2) -> Merge3/1
  Triggered Subsystem7/1(Out1) -> Merge3/2
  [VVMC_VehHoldEnReqAccel_mps2] -> Add10/3
  Constant76/1 -> Switch3/3
  Constant75/1 -> Switch10/3
  Add10/1 -> Divide14/1
  Switch33/1 -> [VVMC_VehHoldDecCtrlBSlope_mps3]  "VVMC_VehHoldDecCtrlBSlope_mps3"
  [VVMC_LastActACCRequiredAccel_mps2] -> Add11/1
  [VVMC_BrkGFBFinal_mps2] -> Add10/2
  Switch9/1 -> Add11/2
  [VVMC_ACCVehHoldReq_flg] -> Timer/1, NOT1/1
  NOT1/1 -> Timer/2
  [task_time_s] -> Timer/3
  Switch13/1 -> Timer/4, Relational Operator30/2
  Timer/1 -> Relational Operator30/1
  Switch34/1 -> [VVMC_VehHoldDecCtrlBEnd_flg]  "VVMC_VehHoldDecCtrlBEnd_flg"
  Constant81/1 -> Switch9/1
  [task_time_s] -> Divide16/2
  [VVMC_VehHoldDecCtrlBSlope_mps3] -> Divide16/1
  Divide16/1 -> Switch9/3
  [VVMC_VehHoldDecCtrlBEnd_flg] -> OR3/2
  [VVMC_ACCVehHoldReq_flg] -> NOT2/1
  NOT2/1 -> OR3/1
  OR3/1 -> Switch9/2
  [VVMC_VehHoldDecCtrlBEnd_flg] -> Timer1/1, NOT3/1
  [task_time_s] -> Timer1/3
  Switch15/1 -> Switch21/3
  Timer1/1 -> Relational Operator32/1
  AND8/1 -> [VVMC_VehHoldDecCtrlHEnd_flg]  "VVMC_VehHoldDecCtrlHEnd_flg"
  Add11/1 -> u2 > 0 (1)6/3
  [VVMC_VehHoldDecCtrlHEnd_flg] -> u2 > 0 (1)6/2
  Constant15/1 -> Switch12/3
  u2 > 0 (1)6/1 -> u2 > 0 (1)5/1  "VVMC_VehHoldDecCtrlAccel_mps2"
  AND6/1 -> Switch8/2
  Constant88/1 -> Switch11/2
  [VVMC_BrkGFB_mps2] -> Switch11/1
  Constant89/1 -> Switch11/3
  Switch11/1 -> [VVMC_BrkGFBFinal_mps2]
  [VVMC_VehHoldDecCtrlHEnd_flg] -> VVMC_VehHoldDecCtrlHEnd_flg/1
  Relational Operator30/1 -> Unit Delay3/1
  [VVMC_ACCVehHoldReq_flg] -> AND8/1
  Relational Operator32/1 -> Unit Delay4/1
  Unit Delay4/1 -> AND7/1
  Constant90/1 -> Relational Operator34/2
  Unit Delay5/1 -> Relational Operator34/1
  Relational Operator34/1 -> OR4/2
  Constant92/1 -> Relational Operator36/2
  Constant91/1 -> Relational Operator35/2
  Relational Operator36/1 -> NOT4/1
  NOT4/1 -> OR5/2
  Relational Operator35/1 -> NOT5/1
  NOT5/1 -> OR5/1
  OR4/1 -> AND3/1
  Constant67/1 -> Relational Operator25/2
  Constant68/1 -> Relational Operator26/2
  [VINP_ACCRequiredAccel_mps2] -> Relational Operator36/1, Relational Operator26/1, Relational Operator25/1, Relational Operator35/1, Unit Delay5/1, Unit Delay2/1
  Relational Operator25/1 -> OR6/1
  Relational Operator26/1 -> OR6/3
  AND7/1 -> AND8/2
  VTQD_FrEDUAvailBrkRgnTq_Nm/1 -> [VTQD_FrEDUAvailBrkRgnTq_Nm]
  [VTQD_FrEDUAvailBrkRgnTq_Nm] -> Add14/2
  Add14/1 -> Relational Operator15/2
  NOT3/1 -> Timer1/2
  VVMC_ACCLowSpdTqCtrl_flg/1 -> [VVMC_ACCLowSpdTqCtrl_flg]
  [VVMC_ACCLowSpdTqCtrl_flg] -> Logical Operator2/3
  [VINP_VehSpeed_kph] -> Relational Operator31/1
  Constant82/1 -> Relational Operator31/2
  Relational Operator31/1 -> Logical Operator2/4
  [VVMC_SPD2ACCAct_flg] -> CMDRepeat/7(VVMC_SPD2ACCAct_flg)
  Constant94/1 -> CMDRepeat/3(TRUE)
  Constant95/1 -> CMDRepeat/4(ZERO_FLOAT)
  [VVMC_AbsDeltaSpd_kph] -> CMDRepeat/1(VVMC_AbsDeltaSpd_kph)
  [VVMC_MeterIndSpeedForCalcu_kph] -> Triggered Subsystem4/1(In1)
  Relational Operator38/1 -> OR6/2
  Constant101/1 -> Relational Operator40/2, Timer2/4
  [task_time_s] -> Timer2/3
  Logical Operator5/1 -> NOT6/1, Timer2/1
  NOT6/1 -> Timer2/2
  Timer2/1 -> Relational Operator40/1
  Relational Operator40/1 -> u2 > 0 (1)7/2
  Constant102/1 -> u2 > 0 (1)7/3
  u2 > 0 (1)7/1 -> Logical Operator2/2
  Constant103/1 -> u2 > 0 (1)7/1
  [VVMC_ActACCRequiredAccel_mps2] -> Relational Operator41/1
  Relational Operator41/1 -> Logical Operator2/6
  Constant104/1 -> Relational Operator41/2
  Constant107/1 -> u2 > 0 (1)8/1
  Constant106/1 -> u2 > 0 (1)8/3
  Relational Operator42/1 -> u2 > 0 (1)8/2
  Timer3/1 -> Relational Operator42/1
  NOT7/1 -> Timer3/2
  Relational Operator18/1 -> NOT7/1, Timer3/1
  [task_time_s] -> Timer3/3
  Constant105/1 -> Timer3/4, Relational Operator42/2
  u2 > 0 (1)8/1 -> Logical Operator2/1
  [VINP_VehSpeed_kph] -> Triggered Subsystem6/1(In1)
  Triggered Subsystem6/1(Out1) -> [VVMC_VehHoldEnSpd_kph]  "VVMC_VehHoldEnSpd_kph"
  Constant38/1 -> Switch3/2
  Switch10/1 -> Divide14/2
  Constant84/1 -> Switch10/2
  Switch3/1 -> Add10/1
  Constant85/1 -> Switch12/2
  Switch12/1 -> u2 > 0 (1)6/1
  [VVMC_VehHoldEnSpd_kph] -> MVMC_VehHoldBDecMap_Y_mps2/1
  MVMC_VehHoldBDecMap_Y_mps2/1 -> Switch3/1
  [VVMC_VehHoldEnSpd_kph] -> MVMC_VehHoldDecCtrlTime_Y_s/1
  MVMC_VehHoldDecCtrlTime_Y_s1/1 -> Switch13/1
  [VVMC_VehHoldEnSpd_kph] -> MVMC_VehHoldDecCtrlTime_Y_s1/1
  Constant87/1 -> Switch13/2
  Constant80/1 -> Switch13/3
  Constant96/1 -> Switch15/2
  [VVMC_VehHoldEnSpd_kph] -> MVMC_VehHoldDecCtrlTime_Y_s2/1
  Constant83/1 -> Switch15/3
  NOT9/1 -> AND9/2
  Relational Operator43/1 -> NOT9/1
  [VINP_VehSpeed_kph] -> Relational Operator43/1
  Constant93/1 -> Relational Operator43/2
  [VVMC_ACCVehHoldReq_flg] -> OR8/3, AND9/1
  AND9/1 -> Switch20/3
  Constant97/1 -> Triggered Subsystem8/1(In1)
  [VVMC_ACCVehHoldReq_flg] -> NOT8/1
  Constant108/1 -> Triggered Subsystem9/1(In1)
  Triggered Subsystem8/1(Out1) -> Merge4/1
  NOT8/1 -> Triggered Subsystem9/Trigger
  Triggered Subsystem9/1(Out1) -> Merge4/2
  Merge4/1 -> [VVMC_ZeroSpdHoldAllow_flg]
  [VVMC_ZeroSpdHoldAllow_flg] -> AND7/2
  VDSC_DISCTurn_flg/1 -> [VDSC_DISCTurn_flg]
  u2 > 0 (3)2/1 -> Relational Operator45/1, Switch16/3, Relational Operator47/1, Switch17/1
  [VDSC_DISCTurn_flg] -> Relational Operator37/1
  Constant109/1 -> Relational Operator37/2
  Relational Operator37/1 -> AND12/1
  Switch17/1 -> Switch16/1
  Constant110/1 -> AND10/2
  Constant111/1 -> Relational Operator44/2
  [VDSC_DISCTurn_flg] -> Relational Operator44/1
  Relational Operator44/1 -> AND11/1
  Relational Operator45/1 -> AND11/2
  Constant112/1 -> Relational Operator45/2
  AND11/1 -> NOT11/1, Timer4/1
  NOT11/1 -> Timer4/2
  [task_time_s] -> Timer4/3
  Constant113/1 -> Timer4/4
  Timer4/1 -> [VVMC_DISCTurnAccTimer_s]
  [VVMC_DISCTurnAccTimer_s] -> Relational Operator46/1
  Constant114/1 -> Relational Operator46/2
  Relational Operator46/1 -> Switch17/2
  AND10/1 -> Switch16/2
  Relational Operator47/1 -> AND12/2
  Constant115/1 -> Relational Operator47/2
  AND12/1 -> AND10/1
  [VVMC_DISCTurnAccTimer_s] -> MVMC_DISCTrunAccJerk_Y_mps3/1
  [VVMC_LastDISCReqAcc_mps2] -> Add6/2
  MVMC_DISCTrunAccJerk_Y_mps3/1 -> Divide3/1
  [VVMC_DISCTurnAccTimer_s] -> MVMC_DISCTrunAccLimit_Y_mps2/1
  MVMC_DISCTrunAccLimit_Y_mps2/1 -> Min/1
  Add6/1 -> Min/2
  Min/1 -> Switch17/3
  [task_time_s] -> Divide3/2
  Divide3/1 -> Add6/1
  VINP_GRADE_Deg/1 -> [VINP_GRADE_Deg]
  Sin2/1 -> Abs3/1
  Degrees to Radians2/1 -> Cast To Single2/1
  Cast To Single2/1 -> Sin2/1
  [VINP_GRADE_Deg] -> Degrees to Radians2/1
  Abs3/1 -> Max/1
  Max/1 -> Relational Operator29/1, Switch8/1
  MVMC_VehHoldDecCtrlTime_Y_s/1 -> Switch10/1
  Switch20/1 -> Triggered Subsystem8/Trigger
  Constant118/1 -> Switch20/2
  MVMC_VehHoldDecCtrlTime_Y_s2/1 -> Switch15/1
  OR8/1 -> Switch20/1
  [VVMC_LastActACCRequiredAccel_mps2] -> Switch12/1
  VINP_LFWhlRotDir_enum/1 -> [VINP_LFWhlRotDir_enum]
  VINP_LRWhlRotDir_enum/1 -> [VINP_LRWhlRotDir_enum]
  VINP_RFWhlRotDir_enum/1 -> [VINP_RFWhlRotDir_enum]
  VINP_RRWhlRotDir_enum/1 -> [VINP_RRWhlRotDir_enum]
  [VINP_LFWhlRotDir_enum] -> Relational Operator49/1
  Constant117/1 -> Relational Operator49/2
  Constant122/1 -> Relational Operator50/2
  [VINP_LRWhlRotDir_enum] -> Relational Operator50/1
  Constant123/1 -> Relational Operator51/2
  [VINP_RFWhlRotDir_enum] -> Relational Operator51/1
  [VINP_RRWhlRotDir_enum] -> Relational Operator52/1
  Constant124/1 -> Relational Operator52/2
  Relational Operator49/1 -> Switch14/2
  Constant125/1 -> Switch14/3
  Constant126/1 -> Switch14/1
  Constant128/1 -> Switch23/1
  Constant127/1 -> Switch23/3
  Relational Operator50/1 -> Switch23/2
  Relational Operator51/1 -> Switch24/2
  Constant129/1 -> Switch24/3
  Constant130/1 -> Switch24/1
  Constant132/1 -> Switch25/1
  Constant131/1 -> Switch25/3
  Relational Operator52/1 -> Switch25/2
  Switch25/1 -> Add12/4
  Switch24/1 -> Add12/3
  Switch23/1 -> Add12/2
  Switch14/1 -> Add12/1
  Add12/1 -> Switch26/2
  Constant133/1 -> Switch26/1
  Constant134/1 -> Switch26/3
  Switch26/1 -> [VVMC_WhlStandstill_flg]
  Switch31/1 -> [VVMC_WhlBackward_flg]
  Constant148/1 -> Switch31/3
  Constant147/1 -> Switch31/1
  Add13/1 -> Switch31/2
  Switch27/1 -> Add13/1
  Switch28/1 -> Add13/2
  Switch29/1 -> Add13/3
  Switch30/1 -> Add13/4
  Relational Operator56/1 -> Switch30/2
  Constant145/1 -> Switch30/3
  Constant146/1 -> Switch30/1
  Constant144/1 -> Switch29/1
  Constant143/1 -> Switch29/3
  Relational Operator55/1 -> Switch29/2
  Relational Operator54/1 -> Switch28/2
  Constant141/1 -> Switch28/3
  Constant142/1 -> Switch28/1
  Constant140/1 -> Switch27/1
  Constant139/1 -> Switch27/3
  Relational Operator53/1 -> Switch27/2
  Constant138/1 -> Relational Operator56/2
  [VINP_RRWhlRotDir_enum] -> Relational Operator56/1
  [VINP_RFWhlRotDir_enum] -> Relational Operator55/1
  Constant137/1 -> Relational Operator55/2
  [VINP_LRWhlRotDir_enum] -> Relational Operator54/1
  Constant136/1 -> Relational Operator54/2
  Constant135/1 -> Relational Operator53/2
  [VINP_LFWhlRotDir_enum] -> Relational Operator53/1
  OR7/1 -> OR8/1
  [VVMC_WhlStandstill_flg] -> OR7/2
  [VVMC_WhlBackward_flg] -> OR7/3
  VVMC_ACCObjDist_m/1 -> [VVMC_ACCObjDist_m]
  [VVMC_ACCObjDist_m] -> Relational Operator48/1
  Relational Operator48/1 -> OR7/1
  Constant119/1 -> Relational Operator48/2
  Divide14/1 -> Switch33/3
  Switch18/1 -> Switch33/1
  Relational Operator57/1 -> AND15/1
  Unit Delay3/1 -> Switch34/3
  VINP_MCPressure_bar/1 -> [VINP_MCPressure_bar]
  [VINP_MCPressure_bar] -> Relational Operator57/1
  [VVMC_VehHoldMCPPass_flg] -> Switch34/1
  Constant154/1 -> Triggered Subsystem10/1(In1)
  Constant153/1 -> Triggered Subsystem11/1(In1)
  NOT10/1 -> Triggered Subsystem11/Trigger
  Triggered Subsystem10/1(Out1) -> Merge5/1
  Triggered Subsystem11/1(Out1) -> Merge5/2
  AND15/1 -> Triggered Subsystem10/Trigger
  Merge5/1 -> [VVMC_VehHoldMCPPass_flg]
  [VINP_GRADE_Deg] -> Max5/1
  [VVMC_EstSlope_Deg] -> Max5/2
  MVMC_VehHoldMCPPass_Y_bar/1 -> Add15/1
  Max5/1 -> MVMC_VehHoldMCPPass_Y_bar/1
  [VVMC_LastADASWhlTqReq_Nm] -> Relational Operator58/1
  Constant155/1 -> Relational Operator58/2
  Relational Operator58/1 -> Switch35/2
  Constant156/1 -> Switch35/1
  Constant157/1 -> Switch35/3
  Switch35/1 -> Add15/2
  Add15/1 -> Relational Operator57/2
  [VVMC_VehHoldDecCtrlCalSW2_flg] -> Switch34/2
  [VVMC_VehHoldDecCtrlCalSW2_flg] -> Switch33/2
  Max4/1 -> Relational Operator61/1
  Constant161/1 -> Triggered Subsystem12/1(In1)
  AND18/1 -> Triggered Subsystem12/Trigger
  NOT12/1 -> Triggered Subsystem13/Trigger
  Detect Increase5/1 -> AND18/4
  Constant149/1 -> Relational Operator61/2
  [VVMC_EstSlope_Deg] -> Max4/2
  Constant150/1 -> Triggered Subsystem13/1(In1)
  [VVMC_ACCVehHoldReq_flg] -> NOT12/1
  Relational Operator61/1 -> AND18/2
  Triggered Subsystem12/1(Out1) -> Merge6/1
  [VINP_GRADE_Deg] -> Max4/1
  [VVMC_ACCVehHoldReq_flg] -> Detect Increase5/1
  Merge6/1 -> [VVMC_VehHoldDecCtrlCalSW2_flg]  "VVMC_VehHoldDecCtrlCalSW2_flg"
  Triggered Subsystem13/1(Out1) -> Merge6/2
  Constant121/1 -> AND18/3
  [VVMC_ACCVehHoldReq_flg] -> AND15/2, NOT10/1
  Constant152/1 -> Relational Operator59/2
  [VVMC_FeatArbitrSta_enum] -> Relational Operator59/1
  Relational Operator59/1 -> u2 > 0 (1)9/2
  [VINP_ACCRequiredAccel_mps2] -> u2 > 0 (1)9/1
  u2 > 0 (1)5/1 -> u2 > 0 (1)9/3
  VVMC_AccelTurnHold_flg/1 -> [VVMC_AccelTurnHold_flg]
  [VVMC_AccelTurnHold_flg] -> NOT14/1
  NOT14/1 -> OR9/2
  [VVMC_VehHoldDecCtrlCalSW2_flg] -> Switch21/2
  Switch21/1 -> Timer1/4, Relational Operator32/2
  Constant162/1 -> Switch21/1
  [VVMC_ActACCRequiredAccel_mps2] -> Unit Delay9/1
  Relational Operator62/1 -> OR8/2
  Constant163/1 -> Relational Operator62/2
  Unit Delay9/1 -> Relational Operator62/1
  Constant86/1 -> Relational Operator33/2
  [VINP_ADASACCSta_enum] -> Relational Operator33/1
  Relational Operator33/1 -> AND3/2
  [VINP_ADASACCSta_enum] -> Relational Operator38/1
  Constant99/1 -> Relational Operator38/2
  OR9/1 -> AND18/1
  Constant98/1 -> OR9/1
  [VVMC_AccelTurnHold_flg] -> Switch18/2
  Constant151/1 -> Switch18/3
  Constant100/1 -> Switch18/1

== system vmc/VMC/VMC/SPD2ACC/SPD2ACC Active Determination ==
  VVMC_FeatArbitrSta_enum : Inport
  Constant : Constant  Value=TRUE
  Constant1 : Constant  Value=FALSE
  Constant13 : Constant  Value=ENUM_FEATARBITRSTA_DISC
  Constant2 : Constant  Value=ENUM_FEATARBITRSTA_ACCDISC
  Constant3 : Constant  Value=ENUM_FEATARBITRSTA_CC
  Constant4 : Constant  Value=ENUM_FEATARBITRSTA_MSA
  SPD2ACC Active Determination : Stateflow chart  TreatAsAtomicUnit=on
  VVMC_SPD2ACCAct_flg : Outport
  wires:
  Constant2/1 -> SPD2ACC Active Determination/5(ENUM_FEATARBITRSTA_ACCDISC)
  Constant13/1 -> SPD2ACC Active Determination/4(ENUM_FEATARBITRSTA_DISC)
  Constant1/1 -> SPD2ACC Active Determination/3(FALSE)
  Constant/1 -> SPD2ACC Active Determination/2(TURE)
  [VVMC_SPD2ACCAct_flg] -> VVMC_SPD2ACCAct_flg/1
  SPD2ACC Active Determination/1(VVMC_SPD2ACCAct_flg) -> [VVMC_SPD2ACCAct_flg]
  [VVMC_FeatArbitrSta_enum] -> SPD2ACC Active Determination/1(VVMC_FeatArbitrSta_enum)
  VVMC_FeatArbitrSta_enum/1 -> [VVMC_FeatArbitrSta_enum]
  Constant3/1 -> SPD2ACC Active Determination/6(ENUM_FEATARBITRSTA_CC)
  Constant4/1 -> SPD2ACC Active Determination/7(ENUM_FEATARBITRSTA_MSA)

== system vmc/VMC/VMC/SafetyControl/Estimate Slope ==
  VINP_LongAccel_Gps : Inport
  VINP_VehSpeed_kph : Inport  Port=2
  VINP_GRADE_deg : Inport  Port=3
  Add : Sum  Inputs=+-
  Asin : Trigonometry  Operator=asin
  Constant1 : Constant  Value=KVMC_EstSlopeLongAccelTs_c
  Constant2 : Constant  Value=KVMC_EstSlopeVehSpdTs_c
  Constant3 : Constant  Value=KVMC_EstSlopeTs_c
  Constant4 : Constant  Value=KVMC_EstSlopeSW_flg
  Constant{5..8} (4 alike) : Constant  Value=C_TASK_10MS_S
  FirstOrderFilter : hcu_lib/Basic_Blocks/FirstOrderFilter
  FirstOrderFilter1 : hcu_lib/Basic_Blocks/FirstOrderFilter
  FirstOrderFilter2 : hcu_lib/Basic_Blocks/FirstOrderFilter
  Gain : Gain  Gain=KPH2MPS
  Gain1 : Gain  Gain=1/GRAVITY_G
  Gain2 : Gain  Gain=RAD2DEG
  Switch : Switch  Criteria=u2 > Threshold
  derivative : hcu_lib/Basic_Blocks/derivative
  VVMC_EstSlope_Deg : Outport
  wires:
  VINP_VehSpeed_kph/1 -> FirstOrderFilter1/1
  Gain/1 -> derivative/1
  VINP_LongAccel_Gps/1 -> FirstOrderFilter/1
  Gain1/1 -> Add/2
  Add/1 -> Asin/1  "sum"
  FirstOrderFilter/1 -> Add/1
  FirstOrderFilter1/1 -> Gain/1
  derivative/1 -> Gain1/1
  Asin/1 -> Gain2/1
  Gain2/1 -> FirstOrderFilter2/1
  FirstOrderFilter2/1 -> Switch/1
  Switch/1 -> VVMC_EstSlope_Deg/1  "VVMC_EstSlopeCal_Deg"
  Constant5/1 -> FirstOrderFilter/2
  Constant1/1 -> FirstOrderFilter/3
  Constant7/1 -> FirstOrderFilter2/2
  Constant3/1 -> FirstOrderFilter2/3
  Constant2/1 -> FirstOrderFilter1/3
  Constant6/1 -> FirstOrderFilter1/2
  Constant4/1 -> Switch/2
  VINP_GRADE_deg/1 -> Switch/3
  Constant8/1 -> derivative/2

== system vmc/VMC/VMC/SafetyControl/LatAccRollingAverage ==
  VINP_LatAccel_Gps : Inport
  Constant3 : Constant  Value=ONE_INT
  Constant4 : Constant  Value=ZERO_FLOAT
  Constant5 : Constant  Value=KVMC_LatAccRollAveLevel_enum
  RollingAverage : Stateflow chart  TreatAsAtomicUnit=on
  VVMC_LatAccRollAve_Gps : Outport
  wires:
  RollingAverage/1(VVMC_LatAccRollAve_Gps) -> [VVMC_LatAccRollAve_Gps]
  VINP_LatAccel_Gps/1 -> [VINP_LatAccel_Gps]
  [VVMC_LatAccRollAve_Gps] -> VVMC_LatAccRollAve_Gps/1
  Constant5/1 -> RollingAverage/1(KVMC_LatAccRollAveLevel_enum)
  Constant3/1 -> RollingAverage/3(ONE_INT)
  Constant4/1 -> RollingAverage/2(ZERO_FLOAT)
  [VINP_LatAccel_Gps] -> RollingAverage/4(VINP_LatAccel_Gps)

== system vmc/VMC/VMC/SafetyControl/Lateral_Module ==
  note: I/O Area
  VINP_VehSpeed_kph : Inport
  VINP_SASAngle_deg : Inport  Port=2
  Lateral_Reference_Model : Subsystem
  VVMC_TheoYawRate_degps : Outport
  wires:
  [VVMC_TheoYawRate_degps] -> VVMC_TheoYawRate_degps/1  "VVMC_TheoYawRate_degps"
  VINP_VehSpeed_kph/1 -> [VINP_VehSpeed_kph]
  Lateral_Reference_Model/1(VVMC_TheoYawRate_degps) -> [VVMC_TheoYawRate_degps]
  VINP_SASAngle_deg/1 -> [VINP_SASAngle_deg]
  [VINP_VehSpeed_kph] -> Lateral_Reference_Model/1(VINP_VehSpeed_kph)
  [VINP_SASAngle_deg] -> Lateral_Reference_Model/2(VINP_SASAngle_deg)
